simulink model "s_heli3d_with_LQ_controller_with_integral"  (Simulink 7.7)
settings: Solver=ode1  StartTime=0.0  StopTime=69  FixedStep=0.007  RelTol=1e-3
values from neighbouring files (symbols this model uses):
  A = double(subs(J_a,{'x1','x2','x3','x4','x5','x6','u1','u2'},{x0(1),x0(2),x0(3),x0(4),x0(5),x0(6),u0(1),u0(2)}))    [linnlsys.m]    (also in o_lqi.m = A_lin)
  B = double(subs(J_b,{'x1','x2','x3','x4','x5','x6','u1','u2'},{x0(1),x0(2),x0(3),x0(4),x0(5),x0(6),u0(1),u0(2)}))    [linnlsys.m]    (also in o_lqi.m = B_lin)
  CMD_RATE_LIMIT = 45.0 * pi / 180    (= 0.785398163397)    [setup_lab_heli_3d.m]    (also in setup_lab_heli_3d_simple.m; setup_lab_heli_3d_various_controler.m; setup_lab_heli_3d_various_controler_with_Kalman_Filter.m)
  K_AMP = 3    [setup_lab_heli_3d.m]    (also in setup_lab_heli_3d_simple.m; setup_lab_heli_3d_various_controler.m; setup_lab_heli_3d_various_controler_with_Kalman_Filter.m)
  L = lqr( Ae, Be, Q, R )    [o_lqi.m]    (also in setup_lab_heli_3d_various_controler.m = Le(:,1:6); setup_lab_heli_3d_various_controler_with_Kalman_Filter.m = lqr( A, B, Q, R ))
  Li = L(:,end-size(C,1)+1:end)    [o_lqi.m]    (also in setup_lab_heli_3d_various_controler.m = Le(:,7:9); setup_lab_heli_3d_various_controler_with_Kalman_Filter.m = Le(:,7:9))
  SAT_INT_ERR_TRAVEL = 7.5    [setup_lab_heli_3d.m]    (also in setup_lab_heli_3d_simple.m; setup_lab_heli_3d_various_controler.m; setup_lab_heli_3d_various_controler_with_Kalman_Filter.m)
  VMAX_AMP = 24    [setup_lab_heli_3d.m]    (also in setup_lab_heli_3d_simple.m; setup_lab_heli_3d_various_controler.m; setup_lab_heli_3d_various_controler_with_Kalman_Filter.m)
  VMAX_DAC = 10    [setup_lab_heli_3d.m]    (also in setup_lab_heli_3d_simple.m; setup_lab_heli_3d_various_controler.m; setup_lab_heli_3d_various_controler_with_Kalman_Filter.m)
libraries: simulink_extras x3
settings Model: Creator=MLevis  LastModifiedBy=signaler  ExtModeTrigDuration=5000  ExtModeArmWhenConnect=off  BufferReuse=off
settings SolverCC: PositivePriorityOrder=on
settings OptimizationCC: BooleanDataType=off  InlineInvariantSignals=on  OptimizeBlockIOStorage=off  BufferReuse=off  ExpressionFolding=off  LocalBlockOutputs=off  InitFltsAndDblsToZero=on
settings DebuggingCC: SaveWithParameterizedLinksMsg=none  SignalResolutionControl=TryResolveAllWithWarning  MultiTaskDSMMsg=warning  MultiTaskCondExecSysMsg=none  StrictBusMsg=Warning
settings RTWCC: SystemTargetFile=quarc_windows.tlc  TemplateMakefile=quarc_default_tmf  Description=QUARC Win32 Target  ProcessScript=quarc_windows_make_rtw_hook  IncludeERTFirstTime=on
settings STFCustomTargetCC: TargetFcnLib=ansi_tfl_tmw.mat  TargetPreCompLibLocation=C:\PROGRA~3\QUARC\lib\2011a\windows\release  FunctionExecutionProfile=off  GeneratePreprocessorConditionals=Disable all  SystemTargetFile=quarc_windows.tlc
settings GRTTargetCC: TargetFcnLib=ansi_tfl_tmw.mat  TargetPreCompLibLocation=C:\PROGRA~3\QUARC\lib\2011a\windows\release  ParMdlRefBuildCompliant=off  CompOptLevelCompliant=off  MatFileLogging=off  ExtMode=on  ExtModeMexFile=quarc_comm

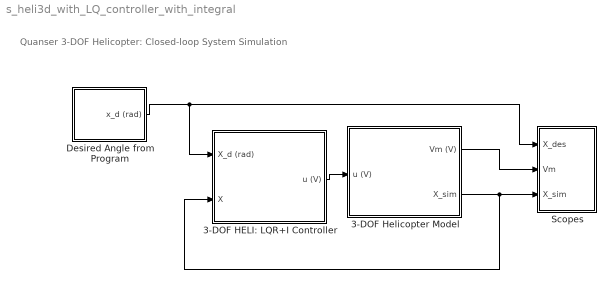
== system s_heli3d_with_LQ_controller_with_integral ==
  note: Quanser 3-DOF Helicopter:
      | Closed-loop System Simulation
  3-DOF HELI: LQR+I Controller : Subsystem  AncestorBlock=heli_2d_lib/2DOF HELI: FF+LQR+I Controller
  3-DOF Helicopter Model : Subsystem
  Desired Angle from Program : Subsystem
  Scopes : Subsystem
  wires:
  Desired Angle from Program/1(x_d (rad)) -> Scopes/1(X_des), 3-DOF HELI: LQR+I Controller/1(X_d (rad))
  3-DOF HELI: LQR+I Controller/1(u (V)) -> 3-DOF Helicopter Model/1(u (V))
  3-DOF Helicopter Model/2(X_sim) -> Scopes/3(X_sim), 3-DOF HELI: LQR+I Controller/2(X)
  3-DOF Helicopter Model/1(Vm (V)) -> Scopes/2(Vm)

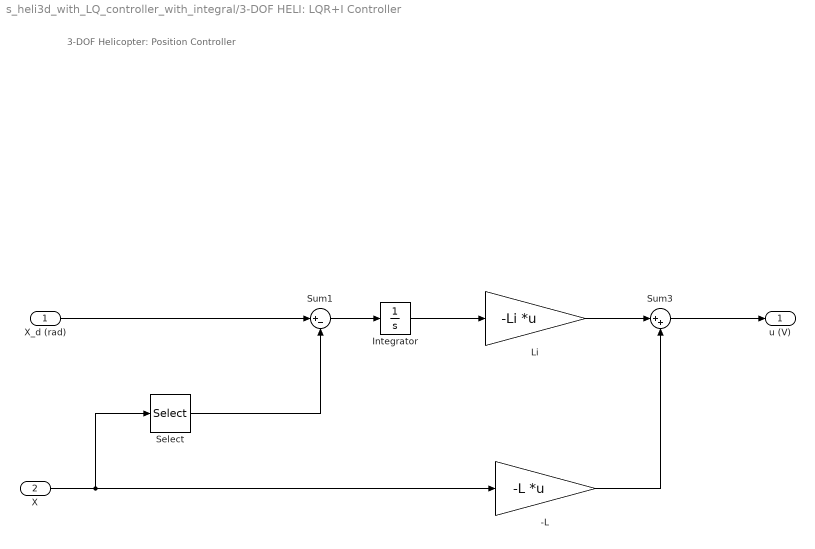
== system s_heli3d_with_LQ_controller_with_integral/3-DOF HELI: LQR+I Controller ==
  note: 3-DOF Helicopter: Position Controller
  X_d (rad) : Inport
  X : Inport  Port=2
  -L : Gain  Gain=-L  Multiplication=Matrix(K*u)
  Integrator : Integrator  LimitOutput=on  UpperSaturationLimit=SAT_INT_ERR_TRAVEL  LowerSaturationLimit=-SAT_INT_ERR_TRAVEL
  Li : Gain  Gain=-Li  Multiplication=Matrix(K*u)
  Select : Selector  InputPortWidth=6  IndexOptions=Index vector (dialog)  Indices=[1:3]  OutputSizes=1
  Sum1 : Sum  Inputs=|+-
  Sum3 : Sum  Inputs=|++
  u (V) : Outport
  wires:
  Li/1 -> Sum3/1
  -L/1 -> Sum3/2
  Sum3/1 -> u (V)/1
  X_d (rad)/1 -> Sum1/1
  Integrator/1 -> Li/1
  Sum1/1 -> Integrator/1
  X/1 -> -L/1, Select/1
  Select/1 -> Sum1/2

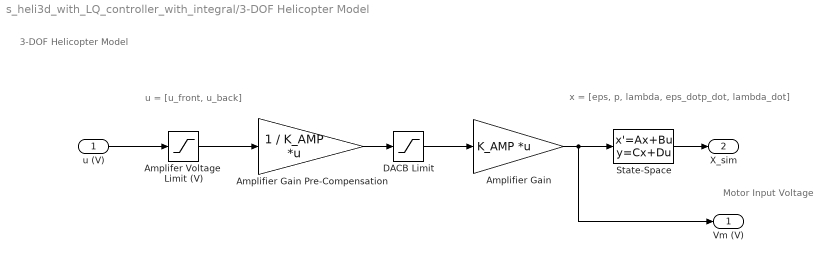
== system s_heli3d_with_LQ_controller_with_integral/3-DOF Helicopter Model ==
  note: x = [eps, p, lambda, eps_dotp_dot, lambda_dot]
  note: u = [u_front, u_back]
  note: Motor Input Voltage
  note: 3-DOF Helicopter Model
  u (V) : Inport
  Amplifer Voltage  Limit (V) : Saturate  UpperLimit=VMAX_AMP  LowerLimit=-VMAX_AMP
  Amplifier Gain : Gain  Gain=K_AMP  Multiplication=Matrix(K*u)  SaturateOnIntegerOverflow=on  OutDataTypeStr=Inherit: Same as input  ParamDataTypeStr=Inherit: Same as input
  Amplifier Gain Pre-Compensation : Gain  Gain=1 / K_AMP  Multiplication=Matrix(K*u)  SaturateOnIntegerOverflow=on  OutDataTypeStr=Inherit: Same as input  ParamDataTypeStr=Inherit: Same as input
  DACB Limit : Saturate  UpperLimit=VMAX_DAC  LowerLimit=-VMAX_DAC
  State-Space : StateSpace  A=A  B=B  C=eye(6,6)  D=zeros(6,2)
  Vm (V) : Outport
  X_sim : Outport  Port=2
  wires:
  u (V)/1 -> Amplifer Voltage  Limit (V)/1
  Amplifier Gain/1 -> Vm (V)/1, State-Space/1
  State-Space/1 -> X_sim/1
  Amplifer Voltage  Limit (V)/1 -> Amplifier Gain Pre-Compensation/1
  Amplifier Gain Pre-Compensation/1 -> DACB Limit/1
  DACB Limit/1 -> Amplifier Gain/1

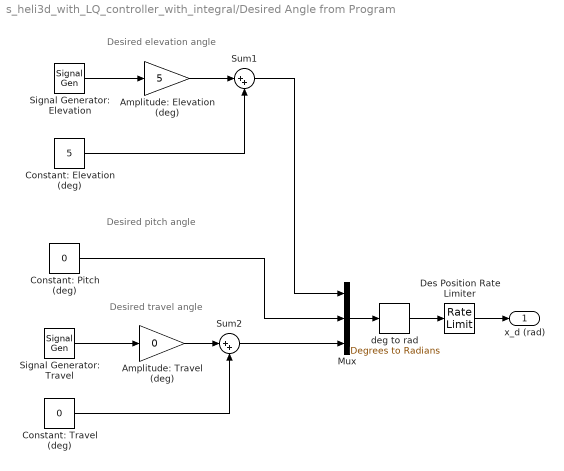
== system s_heli3d_with_LQ_controller_with_integral/Desired Angle from Program ==
  note: Desired elevation angle
  note: Desired travel angle
  note: Desired pitch angle
  Amplitude: Elevation (deg) : Gain  Gain=5
  Amplitude: Travel (deg) : Gain  Gain=0
  Constant: Elevation (deg) : Constant  Value=5
  Constant: Pitch (deg) : Constant  Value=0
  Constant: Travel (deg) : Constant  Value=0
  Des Position Rate Limiter : RateLimiter  RisingSlewLimit=CMD_RATE_LIMIT  FallingSlewLimit=-CMD_RATE_LIMIT  SampleTimeMode=inherited
  Mux : Mux  Inputs=3
  Signal Generator: Elevation : SignalGenerator  WaveForm=square  Frequency=0.02
  Signal Generator: Travel : SignalGenerator  WaveForm=square  Frequency=0.02
  Sum1 : Sum  Inputs=|++
  Sum2 : Sum  Inputs=|++
  deg to rad : simulink_extras/Transformations/Degrees to Radians  SystemSampleTime=-1
  x_d (rad) : Outport
  wires:
  Mux/1 -> deg to rad/1
  Constant: Elevation (deg)/1 -> Sum1/2
  Amplitude: Elevation (deg)/1 -> Sum1/1
  Signal Generator: Elevation/1 -> Amplitude: Elevation (deg)/1
  Constant: Travel (deg)/1 -> Sum2/2
  Amplitude: Travel (deg)/1 -> Sum2/1
  Signal Generator: Travel/1 -> Amplitude: Travel (deg)/1
  Sum2/1 -> Mux/3
  deg to rad/1 -> Des Position Rate Limiter/1
  Constant: Pitch (deg)/1 -> Mux/2
  Sum1/1 -> Mux/1
  Des Position Rate Limiter/1 -> x_d (rad)/1

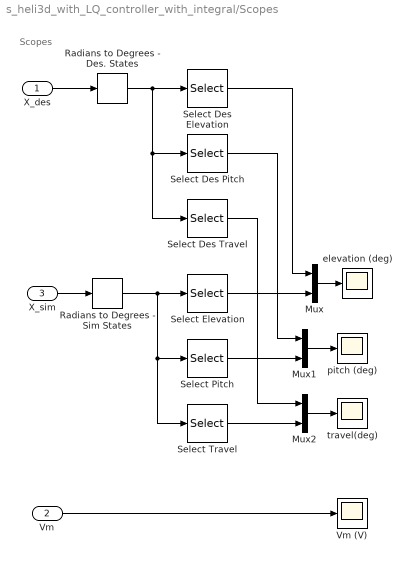
== system s_heli3d_with_LQ_controller_with_integral/Scopes ==
  note: Scopes
  X_des : Inport
  Vm : Inport  Port=2
  X_sim : Inport  Port=3
  Mux : Mux  Inputs=2
  Mux1 : Mux  Inputs=2
  Mux2 : Mux  Inputs=2
  Radians to Degrees - Des. States : simulink_extras/Transformations/Radians to Degrees  SystemSampleTime=-1
  Radians to Degrees - Sim States : simulink_extras/Transformations/Radians to Degrees  SystemSampleTime=-1
  Select Des Elevation : Selector  InputPortWidth=3  IndexOptions=Index vector (dialog)  Indices=1  OutputSizes=1
  Select Des Pitch : Selector  InputPortWidth=3  IndexOptions=Index vector (dialog)  Indices=2  OutputSizes=1
  Select Des Travel : Selector  InputPortWidth=3  IndexOptions=Index vector (dialog)  Indices=3  OutputSizes=1
  Select Elevation : Selector  InputPortWidth=6  IndexOptions=Index vector (dialog)  Indices=1  OutputSizes=1
  Select Pitch : Selector  InputPortWidth=6  IndexOptions=Index vector (dialog)  Indices=2  OutputSizes=1
  Select Travel : Selector  InputPortWidth=6  IndexOptions=Index vector (dialog)  Indices=3  OutputSizes=1
  Vm (V) : Scope
      settings: TickLabels=on  TimeRange=60  YMin=-25  YMax=25  SaveName=ScopeData4  DataFormat=Array
  elevation (deg) : Scope
      settings: TickLabels=on  TimeRange=0.0006524839931785209  YMin=8.999856219450567  YMax=9.000116462070146  DataFormat=Array
  pitch (deg) : Scope
      settings: TickLabels=on  TimeRange=60  YMin=-30  YMax=30  DataFormat=Array
  travel(deg) : Scope
      settings: TickLabels=on  TimeRange=60  YMin=-100  YMax=100  SaveName=ScopeData2  DataFormat=Array
  wires:
  X_des/1 -> Radians to Degrees - Des. States/1
  X_sim/1 -> Radians to Degrees - Sim States/1
  Mux/1 -> elevation (deg)/1
  Mux1/1 -> pitch (deg)/1
  Vm/1 -> Vm (V)/1
  Radians to Degrees - Sim States/1 -> Select Elevation/1, Select Pitch/1, Select Travel/1
  Mux2/1 -> travel(deg)/1
  Select Elevation/1 -> Mux/2
  Select Pitch/1 -> Mux1/2
  Select Travel/1 -> Mux2/2
  Radians to Degrees - Des. States/1 -> Select Des Elevation/1, Select Des Pitch/1, Select Des Travel/1
  Select Des Elevation/1 -> Mux/1
  Select Des Pitch/1 -> Mux1/1
  Select Des Travel/1 -> Mux2/1
